simulink model "w2_prob3_reference_model"  (R2020a)
settings: Solver=ode45  StartTime=0.0  StopTime=10  RelTol=1e-3
undefined symbols (not defined in the file or in its folder): b, ki, kp, m
settings Model: DataDictionary=sonali.sldd  Creator=sonal  LastModifiedBy=sonal
settings DataIOCC: SaveOutput=off  SaveTime=off

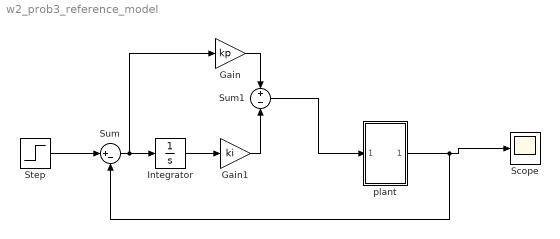
== system w2_prob3_reference_model ==
  Gain : Gain  Gain=kp
  Gain1 : Gain  Gain=ki
  Integrator : Integrator
  Scope : Scope
  Step : Step  Time=0  After=u  SampleTime=0
  Sum : Sum  Inputs=|+-
  Sum1 : Sum  Inputs=+-
  plant : Subsystem
  wires:
  Gain1/1 -> Sum1/2
  Sum/1 -> Integrator/1, Gain/1
  Sum1/1 -> plant/1(In1)
  Integrator/1 -> Gain1/1
  plant/1(Out1) -> Scope/1, Sum/2
  Step/1 -> Sum/1
  Gain/1 -> Sum1/1

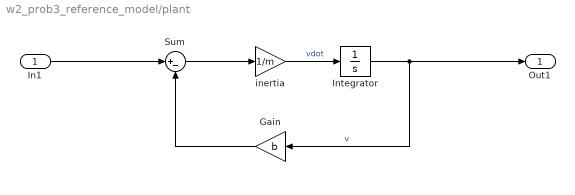
== system w2_prob3_reference_model/plant ==
  In1 : Inport
  Gain : Gain  Gain=b
  Integrator : Integrator
  Sum : Sum  Inputs=|+-
  inertia : Gain  Gain=1/m
  Out1 : Outport
  wires:
  In1/1 -> Sum/1
  Gain/1 -> Sum/2
  inertia/1 -> Integrator/1  "vdot"
  Sum/1 -> inertia/1
  Integrator/1 -> Gain/1, Out1/1  "v"
